simulink model "M2_chart_3_simfun_2"  (R2024a)
settings: Solver=FixedStepDiscrete  StartTime=0.0  StopTime=10.0  FixedStep=0.001  RelTol=1e-3  EnableMultiTasking=on
libraries: simulink x1
settings Model: Creator=saura  LastModifiedBy=Ishant
settings SolverCC: AlgebraicLoopSolver=TrustRegion  AutoInsertRateTranBlk=on
settings DataIOCC: LimitDataPoints=on
settings OptimizationCC: LifeSpan=inf
settings DebuggingCC: UnconnectedInputMsg=warning  UnconnectedOutputMsg=warning  UnconnectedLineMsg=warning  AllowSymbolicDim=off  SFUnexpectedBacktrackingDiag=warning  SFNoUnconditionalDefaultTransitionDiag=warning  SFExecutionAtInitializationDiag=none  ArithmeticOperatorsInVariantConditions=warning
settings ModelReferenceCC: EnableRefExpFcnMdlSchedulingChecks=on
settings SFSimCC: SimUseLocalCustomCode=off  CustomCodeUndefinedFunction=UseInterfaceOnly
settings RTWCC: RTWUseLocalCustomCode=off  GPUComputeCapability=3.5  DLArmComputeVersion=19.05
settings CodeAppCC: StateflowObjectComments=on
settings GRTTargetCC: TargetLangStandard=C89/C90 (ANSI)
settings ConfigComp: CovMetricSettings=dw  CovSaveCumulativeToWorkspaceVar=on  CovSaveSingleToWorkspaceVar=on  CovExternalEMLEnable=off  CovSFcnEnable=off

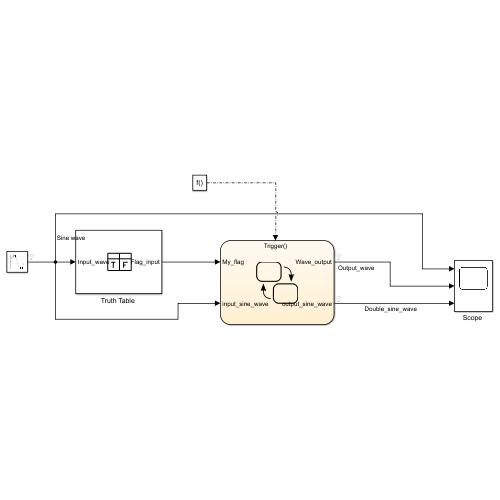
[thumbnail: Simulink's stored preview of the top-level diagram]
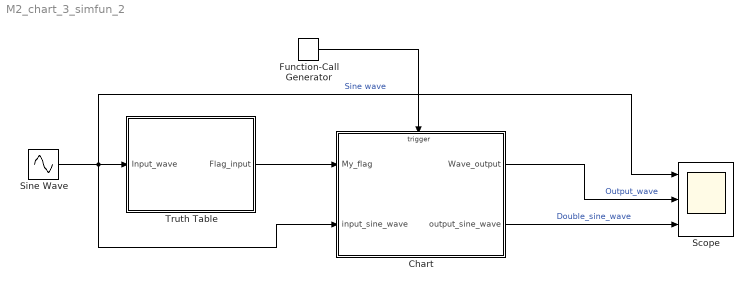
== system M2_chart_3_simfun_2 ==
  Chart : Stateflow chart  TreatAsAtomicUnit=on
  Function-Call Generator : simulink/Ports & Subsystems/Function-Call Generator  sample_time=0.001  numberOfIterations=1  DisallowWideOutput=off
  "Scope " : Scope  NumInputPorts=3
  Sine Wave : Sin  SampleTime=0.001
  "Truth Table " : Truth Table  TreatAsAtomicUnit=on
  wires:
  Sine Wave/1 -> Chart/2(input_sine_wave), "Truth Table "/1(Input_wave), "Scope "/1  "Sine wave"
  "Truth Table "/1(Flag_input) -> Chart/1(My_flag)
  Chart/1(Wave_output) -> "Scope "/2  "Output_wave"
  Chart/2(output_sine_wave) -> "Scope "/3  "Double_sine_wave"
  Function-Call Generator/1 -> Chart/Trigger

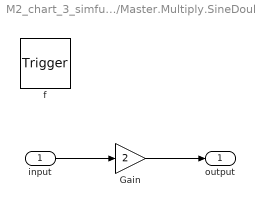
== system M2_chart_3_simfun_2/Chart/Master.Multiply.SineDouble ==
  input : Inport  OutDataTypeStr=double  PortDimensions=1
  f : TriggerPort  TriggerType=function-call  VariantControl=(inherit)
      settings: CopyFcn=Stateflow.SLINSF.SimulinkMan.removeBlockPreDeleteFcn  PreDeleteFcn=Stateflow.SLINSF.SimulinkMan.unsafePredeleteFcn
  Gain : Gain  Gain=2
  output : Outport
  wires:
  Gain/1 -> output/1
  input/1 -> Gain/1

== matlab function M2_chart_3_simfun_2/Truth Table  ==
  data: Input_wave input; Flag_input output
function Flag_input = fcn(Input_wave)

aVarTruthTableCondition_1 = false;
aVarTruthTableCondition_2 = false;


% Output_when_value_less than 0.5

aVarTruthTableCondition_1 = logical(Input_wave<=0.5);

% Output_when_value_Greater than 0.5

aVarTruthTableCondition_2 = logical(Input_wave >0.5);

if (aVarTruthTableCondition_2)
    aFcnTruthTableAction_2();
elseif (aVarTruthTableCondition_1)
    aFcnTruthTableAction_1();
else % Default
    aFcnTruthTableAction_3();
end

function aFcnTruthTableAction_1()

% Example action 1 called from D2 column in condition table

Flag_input = 1;

function aFcnTruthTableAction_2()

% Example action 2 called from D1 column in condition table

Flag_input = -1;

function aFcnTruthTableAction_3()

% Error

Flag_input =0

== stateflow chart M2_chart_3_simfun_2/Chart ==
  state Master
    state Truth_table_IN [parallel]
      en:
      Wave_output=0;
      settings: executionOrder=1
      state On
        en:
        during:
        Wave_output=1;
      state Off
        during:
        Wave_output=-1;
      (default) -> On
      Off -> On : [My_flag==-1]
      On -> Off : [My_flag==1]
    state Multiply [parallel]
      en,during:
      output_sine_wave=SineDouble(input_sine_wave);
      settings: executionOrder=2
      state output=SineDouble(input) [function]
  data: data local; output function_output; input function_input double size=1; Wave_output output double; My_flag input double; input_sine_wave input double size=1; output_sine_wave output double
  events: Trigger input FUNCTION_CALL_EVENT
